simulink model "selmotor6"  (Simulink 2.09)
settings: Solver=VariableStepDiscrete  StartTime=0.0  StopTime=1  FixedStep=0.1  MaxStep=0.01  RelTol=1e-3  AbsTol=1e-6
settings Model: OutputTimes=[1]  SaveTime=off  SaveOutput=off  ConsistencyChecking=off  RTWTemplateMakefile=grt_vc.tmf

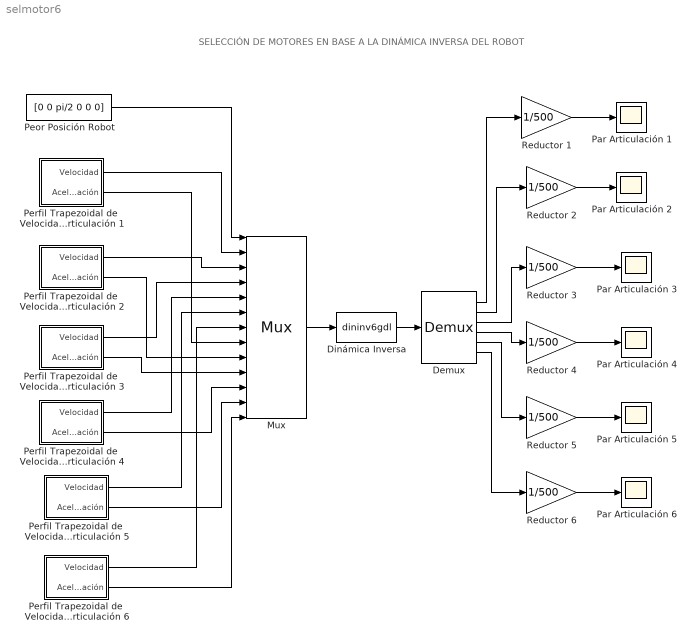
== system selmotor6 ==
  note: SELECCIÓN DE MOTORES EN BASE
      | A LA DINÁMICA INVERSA DEL ROBOT
  Demux : Demux  Outputs=6
  Dinámica Inversa : MATLABFcn  MATLABFcn=dininv6gdl  OutputWidth=6
  Mux : Mux  Inputs=13
  Par Articulación {1..6} (6 alike) : Scope
      Par Articulación 1 settings: TickLabels=on  TimeRange=auto  YMin=-0.075  YMax=0.005  SaveToWorkspace=off  SaveName=ScopeData  LimitMaxRows=off
      Par Articulación 2 settings: TickLabels=on  TimeRange=auto  YMin=-5  YMax=5  SaveToWorkspace=off  SaveName=ScopeData  LimitMaxRows=off
      Par Articulación 3 settings: TickLabels=on  TimeRange=auto  YMin=-5  YMax=5  SaveToWorkspace=off  SaveName=ScopeData  LimitMaxRows=off
      Par Articulación 4 settings: TickLabels=on  TimeRange=auto  YMin=-5  YMax=5  SaveToWorkspace=off  SaveName=ScopeData  LimitMaxRows=off
      Par Articulación 5 settings: TickLabels=on  TimeRange=auto  YMin=-5  YMax=5  SaveToWorkspace=off  SaveName=ScopeData  LimitMaxRows=off
      Par Articulación 6 settings: TickLabels=on  TimeRange=auto  YMin=-5  YMax=5  SaveToWorkspace=off  SaveName=ScopeData  LimitMaxRows=off
  Peor Posición Robot : Constant  Value=[0 0 pi/2 0 0 0]
  Perfil Trapezoidal de  Velocidad Articulación 1 : Subsystem  mask(Perfil Trapezoidal de Velocidad){velmax=pi/3, tacel=0.1, tconst=0.4, tdecel=0.1}
      mask prompts: velmax "Velocidad máxima"; tacel "Tiempo aceleración"; tconst "Tiempo constante"; tdecel "Tiempo deceleración"
  Perfil Trapezoidal de  Velocidad Articulación 2 : Subsystem  mask(Perfil Trapezoidal de Velocidad){velmax=-pi/3, tacel=0.1, tconst=0.4, tdecel=0.1}
      mask prompts: velmax "Velocidad máxima"; tacel "Tiempo aceleración"; tconst "Tiempo constante"; tdecel "Tiempo deceleración"
  Perfil Trapezoidal de  Velocidad Articulación 3 : Subsystem  mask(Perfil Trapezoidal de Velocidad){velmax=-pi/3, tacel=0.1, tconst=0.4, tdecel=0.1}
      mask prompts: velmax "Velocidad máxima"; tacel "Tiempo aceleración"; tconst "Tiempo constante"; tdecel "Tiempo deceleración"
  Perfil Trapezoidal de  Velocidad Articulación 4 : Subsystem  mask(Perfil Trapezoidal de Velocidad){velmax=pi/3, tacel=0.1, tconst=0.4, tdecel=0.1}
      mask prompts: velmax "Velocidad máxima"; tacel "Tiempo aceleración"; tconst "Tiempo constante"; tdecel "Tiempo deceleración"
  Perfil Trapezoidal de  Velocidad Articulación 5 : Subsystem  mask(Perfil Trapezoidal de Velocidad){velmax=-pi/3, tacel=0.1, tconst=0.4, tdecel=0.1}
      mask prompts: velmax "Velocidad máxima"; tacel "Tiempo aceleración"; tconst "Tiempo constante"; tdecel "Tiempo deceleración"
  Perfil Trapezoidal de  Velocidad Articulación 6 : Subsystem  mask(Perfil Trapezoidal de Velocidad){velmax=pi/3, tacel=0.1, tconst=0.4, tdecel=0.1}
      mask prompts: velmax "Velocidad máxima"; tacel "Tiempo aceleración"; tconst "Tiempo constante"; tdecel "Tiempo deceleración"
  Reductor {1..6} (6 alike) : Gain  Gain=1/500
  wires:
  Demux/6 -> Reductor 6/1
  Demux/5 -> Reductor 5/1
  Demux/4 -> Reductor 4/1
  Demux/3 -> Reductor 3/1
  Demux/2 -> Reductor 2/1
  Demux/1 -> Reductor 1/1
  Perfil Trapezoidal de  Velocidad Articulación 6/2(Aceleración) -> Mux/13
  Perfil Trapezoidal de  Velocidad Articulación 5/2(Aceleración) -> Mux/12
  Perfil Trapezoidal de  Velocidad Articulación 4/2(Aceleración) -> Mux/11
  Perfil Trapezoidal de  Velocidad Articulación 3/2(Aceleración) -> Mux/10
  Perfil Trapezoidal de  Velocidad Articulación 2/2(Aceleración) -> Mux/9
  Perfil Trapezoidal de  Velocidad Articulación 1/2(Aceleración) -> Mux/8
  Perfil Trapezoidal de  Velocidad Articulación 6/1(Velocidad) -> Mux/7
  Perfil Trapezoidal de  Velocidad Articulación 5/1(Velocidad) -> Mux/6
  Perfil Trapezoidal de  Velocidad Articulación 4/1(Velocidad) -> Mux/5
  Reductor 6/1 -> Par Articulación 6/1
  Reductor 4/1 -> Par Articulación 4/1
  Reductor 3/1 -> Par Articulación 3/1
  Reductor 2/1 -> Par Articulación 2/1
  Reductor 5/1 -> Par Articulación 5/1
  Perfil Trapezoidal de  Velocidad Articulación 3/1(Velocidad) -> Mux/4
  Perfil Trapezoidal de  Velocidad Articulación 2/1(Velocidad) -> Mux/3
  Perfil Trapezoidal de  Velocidad Articulación 1/1(Velocidad) -> Mux/2
  Reductor 1/1 -> Par Articulación 1/1
  Mux/1 -> Dinámica Inversa/1
  Peor Posición Robot/1 -> Mux/1
  Dinámica Inversa/1 -> Demux/1

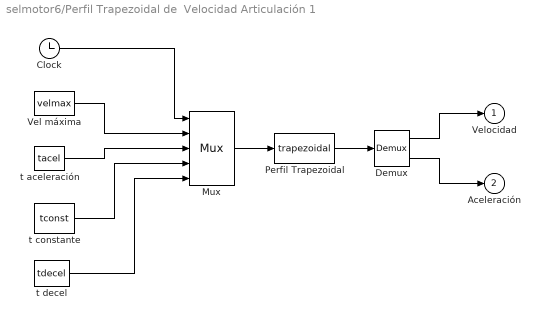
== system selmotor6/Perfil Trapezoidal de  Velocidad Articulación 1 ==
  Clock : Clock
  Demux : Demux  Outputs=2
  Mux : Mux  Inputs=5
  Perfil Trapezoidal : MATLABFcn  MATLABFcn=trapezoidal  OutputWidth=2
  Vel máxima : Constant  Value=velmax
  t aceleración : Constant  Value=tacel
  t constante : Constant  Value=tconst
  t decel : Constant  Value=tdecel
  Velocidad : Outport  Port=1  InitialOutput=0
  Aceleración : Outport  Port=2  InitialOutput=0
  wires:
  Perfil Trapezoidal/1 -> Demux/1
  Demux/2 -> Aceleración/1
  Demux/1 -> Velocidad/1
  Clock/1 -> Mux/1
  Vel máxima/1 -> Mux/2
  t aceleración/1 -> Mux/3
  t constante/1 -> Mux/4
  t decel/1 -> Mux/5
  Mux/1 -> Perfil Trapezoidal/1

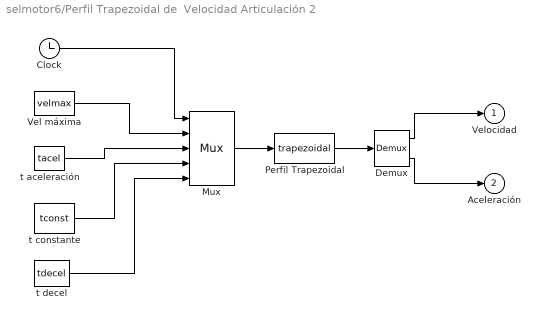
== system selmotor6/Perfil Trapezoidal de  Velocidad Articulación 2 ==
  Clock : Clock
  Demux : Demux  Outputs=2
  Mux : Mux  Inputs=5
  Perfil Trapezoidal : MATLABFcn  MATLABFcn=trapezoidal  OutputWidth=2
  Vel máxima : Constant  Value=velmax
  t aceleración : Constant  Value=tacel
  t constante : Constant  Value=tconst
  t decel : Constant  Value=tdecel
  Velocidad : Outport  Port=1  InitialOutput=0
  Aceleración : Outport  Port=2  InitialOutput=0
  wires:
  Mux/1 -> Perfil Trapezoidal/1
  t decel/1 -> Mux/5
  t constante/1 -> Mux/4
  t aceleración/1 -> Mux/3
  Vel máxima/1 -> Mux/2
  Clock/1 -> Mux/1
  Demux/1 -> Velocidad/1
  Demux/2 -> Aceleración/1
  Perfil Trapezoidal/1 -> Demux/1

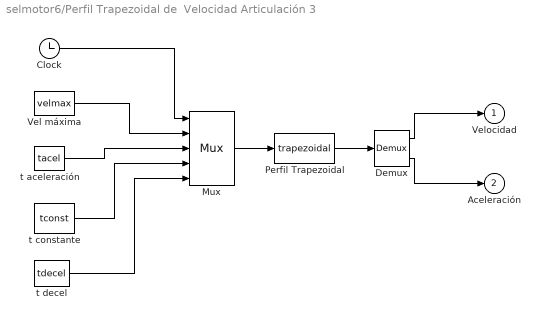
== system selmotor6/Perfil Trapezoidal de  Velocidad Articulación 3 ==
  Clock : Clock
  Demux : Demux  Outputs=2
  Mux : Mux  Inputs=5
  Perfil Trapezoidal : MATLABFcn  MATLABFcn=trapezoidal  OutputWidth=2
  Vel máxima : Constant  Value=velmax
  t aceleración : Constant  Value=tacel
  t constante : Constant  Value=tconst
  t decel : Constant  Value=tdecel
  Velocidad : Outport  Port=1  InitialOutput=0
  Aceleración : Outport  Port=2  InitialOutput=0
  wires:
  Mux/1 -> Perfil Trapezoidal/1
  t decel/1 -> Mux/5
  t constante/1 -> Mux/4
  t aceleración/1 -> Mux/3
  Vel máxima/1 -> Mux/2
  Clock/1 -> Mux/1
  Demux/1 -> Velocidad/1
  Demux/2 -> Aceleración/1
  Perfil Trapezoidal/1 -> Demux/1

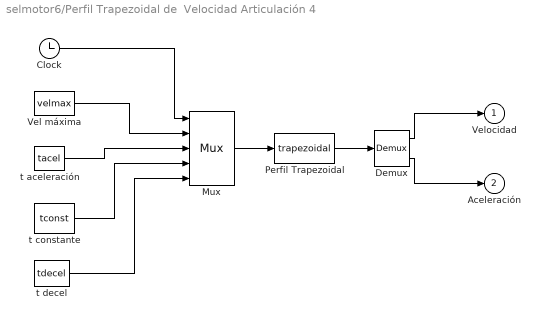
== system selmotor6/Perfil Trapezoidal de  Velocidad Articulación 4 ==
  Clock : Clock
  Demux : Demux  Outputs=2
  Mux : Mux  Inputs=5
  Perfil Trapezoidal : MATLABFcn  MATLABFcn=trapezoidal  OutputWidth=2
  Vel máxima : Constant  Value=velmax
  t aceleración : Constant  Value=tacel
  t constante : Constant  Value=tconst
  t decel : Constant  Value=tdecel
  Velocidad : Outport  Port=1  InitialOutput=0
  Aceleración : Outport  Port=2  InitialOutput=0
  wires:
  Perfil Trapezoidal/1 -> Demux/1
  Demux/2 -> Aceleración/1
  Demux/1 -> Velocidad/1
  Clock/1 -> Mux/1
  Vel máxima/1 -> Mux/2
  t aceleración/1 -> Mux/3
  t constante/1 -> Mux/4
  t decel/1 -> Mux/5
  Mux/1 -> Perfil Trapezoidal/1

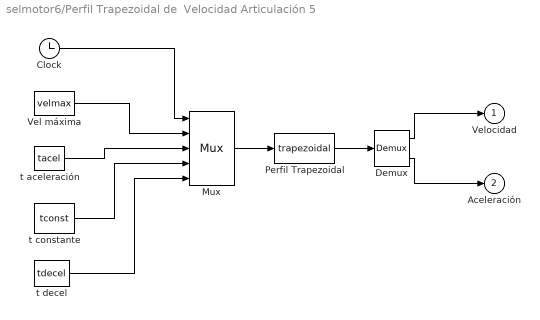
== system selmotor6/Perfil Trapezoidal de  Velocidad Articulación 5 ==
  Clock : Clock
  Demux : Demux  Outputs=2
  Mux : Mux  Inputs=5
  Perfil Trapezoidal : MATLABFcn  MATLABFcn=trapezoidal  OutputWidth=2
  Vel máxima : Constant  Value=velmax
  t aceleración : Constant  Value=tacel
  t constante : Constant  Value=tconst
  t decel : Constant  Value=tdecel
  Velocidad : Outport  Port=1  InitialOutput=0
  Aceleración : Outport  Port=2  InitialOutput=0
  wires:
  Mux/1 -> Perfil Trapezoidal/1
  t decel/1 -> Mux/5
  t constante/1 -> Mux/4
  t aceleración/1 -> Mux/3
  Vel máxima/1 -> Mux/2
  Clock/1 -> Mux/1
  Demux/1 -> Velocidad/1
  Demux/2 -> Aceleración/1
  Perfil Trapezoidal/1 -> Demux/1

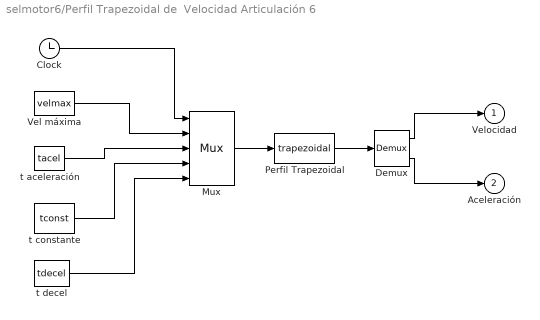
== system selmotor6/Perfil Trapezoidal de  Velocidad Articulación 6 ==
  Clock : Clock
  Demux : Demux  Outputs=2
  Mux : Mux  Inputs=5
  Perfil Trapezoidal : MATLABFcn  MATLABFcn=trapezoidal  OutputWidth=2
  Vel máxima : Constant  Value=velmax
  t aceleración : Constant  Value=tacel
  t constante : Constant  Value=tconst
  t decel : Constant  Value=tdecel
  Velocidad : Outport  Port=1  InitialOutput=0
  Aceleración : Outport  Port=2  InitialOutput=0
  wires:
  Perfil Trapezoidal/1 -> Demux/1
  Demux/2 -> Aceleración/1
  Demux/1 -> Velocidad/1
  Clock/1 -> Mux/1
  Vel máxima/1 -> Mux/2
  t aceleración/1 -> Mux/3
  t constante/1 -> Mux/4
  t decel/1 -> Mux/5
  Mux/1 -> Perfil Trapezoidal/1
